simulink model "waterTankProcess_model_continuous_fullOrderObserver"  (R2017a)
settings: Solver=ode4  StartTime=0.0  StopTime=SIM_TIME  FixedStep=STEP_SIZE  RelTol=1e-3  EnableMultiTasking=on
values from neighbouring files (symbols this model uses):
  At = 0.785    [TwoTankSystem.m]
  Av0 = 0.0122    [TwoTankSystem.m]
  Av1 = 1.2*0.0122    (= 0.01464)    [TwoTankSystem.m]
  B = B(:,1:2)    [TwoTankSystem.m]
  C0 = 0.056    [TwoTankSystem.m]
  C1 = [0 kh 0 0;0 0 kt 0;0 0 0 kt]    [TwoTankSystem.m]
  Dv = 2.66    [TwoTankSystem.m]
  ka = 0.004    [TwoTankSystem.m]
  kh = 2    [TwoTankSystem.m]
  kt = 0.1    [TwoTankSystem.m]
  L = place(A',C',lambda_obs_des)'    [TwoTankSystem.m]
  L1 = place(A',C1',lambda_obs_des)'    [TwoTankSystem.m]
  T1 = 3000    [TwoTankSystem.m]
  T2 = 4000    [TwoTankSystem.m]
  Tc = 1500    [TwoTankSystem.m]
  Tc0 = 30    [TwoTankSystem.m]
  Tc1 = 20    [TwoTankSystem.m]
  Tv = 2200    [TwoTankSystem.m]
  Tw = 300    [TwoTankSystem.m]
  Tw0 = 60    [TwoTankSystem.m]
  Tw1 = 75    [TwoTankSystem.m]
  u0 = u0(1:2,1)    [TwoTankSystem.m]
  uc0 = 5    [TwoTankSystem.m]
  uc1 = 3.5    [TwoTankSystem.m]
  uw0 = 5    [TwoTankSystem.m]
  uw1 = 6.5    [TwoTankSystem.m]
  x0 = xFinal'    [TwoTankSystem.m]
  xhat0 = 1.0*x0-x0    [TwoTankSystem.m]
  Y0 = C*x0    [TwoTankSystem.m]
undefined symbols (not defined in the file or in its folder): A, C
settings Model: Creator=roga  LastModifiedBy=Roberto
settings DataIOCC: LimitDataPoints=on  SaveFinalState=on  SaveFormat=Array
settings OptimizationCC: LifeSpan=inf
settings DebuggingCC: UnderspecifiedInitializationDetection=Classic  MergeDetectMultiDrivingBlocksExec=none  SolverPrmCheckMsg=warning  StateNameClashWarn=warning  SFUnexpectedBacktrackingDiag=warning  SFNoUnconditionalDefaultTransitionDiag=warning  SFExecutionAtInitializationDiag=none
settings HardwareCC: ProdBitPerPointer=32  ProdBitPerSizeT=32  ProdBitPerPtrDiffT=32  ProdLargestAtomicFloat=None  ProdIntDivRoundTo=Undefined  ProdEndianess=Unspecified  ProdWordSize=32  ProdHWDeviceType=32-bit Generic
settings ModelReferenceCC: PropagateSignalLabelsOutOfModel=off
settings GRTTargetCC: TargetLangStandard=C89/C90 (ANSI)  GeneratePreprocessorConditionals=Disable all
settings ConfigComp: CovMetricSettings=dw  CovHtmlReporting=on  CovSaveCumulativeToWorkspaceVar=on  CovSaveSingleToWorkspaceVar=on  CovExternalEMLEnable=off

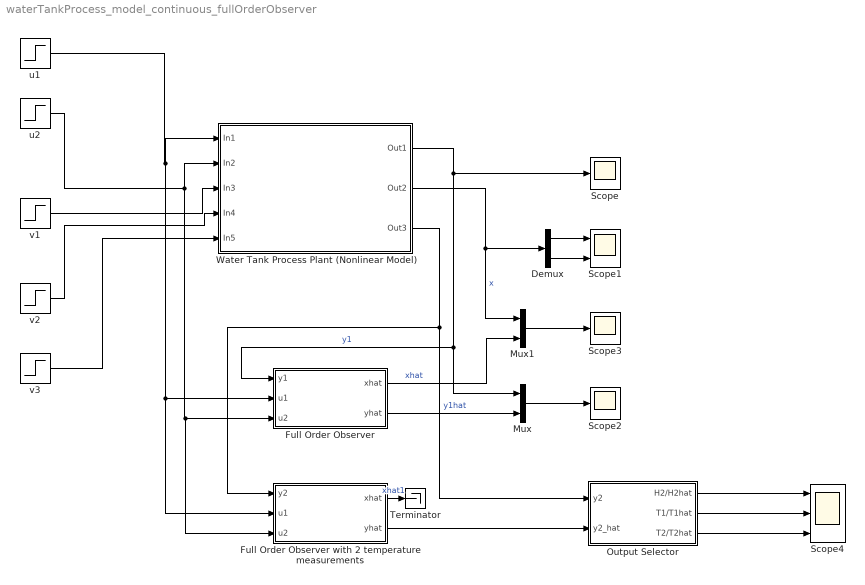
== system waterTankProcess_model_continuous_fullOrderObserver ==
  Demux : Demux  Outputs=2
  Full Order Observer : Subsystem
  Full Order Observer with 2 temperature measurements : Subsystem
  Mux : Mux  Inputs=2
  Mux1 : Mux  Inputs=2
  Output Selector : Subsystem
  Scope : Scope
  Scope1 : Scope  NumInputPorts=2
  Scope2 : Scope
  Scope3 : Scope
  Scope4 : Scope  NumInputPorts=3
  Terminator : Terminator
  Water Tank Process Plant (Nonlinear Model) : Subsystem
      mask Display:
      | port_label('output',1,'y_1','texmode','on')
      | port_label('output',2,'x','texmode','on')
      | port_label('output',3,'y_2','texmode','on')
      | port_label('input',1,'u_1','texmode','on')
      | port_label('input',2,'u_2','texmode','on')
      | port_label('input',3,'A_v','texmode','on')
      | port_label('input',4,'T_w','texmode','on')
      | port_label('input',5,'T_c','texmode','on')
  u1 : Step  Time=Tw  Before=uw0  After=uw1  SampleTime=0
  u2 : Step  Time=Tc  Before=uc0  After=uc1  SampleTime=0
  v1 : Step  Time=Tv  Before=Av0  After=Av1  SampleTime=0
  v2 : Step  Time=T1  Before=Tw0  After=Tw1  SampleTime=0
  v3 : Step  Time=T2  Before=Tc0  After=Tc1  SampleTime=0
  wires:
  Demux/1 -> Scope1/1
  Demux/2 -> Scope1/2
  u1/1 -> Full Order Observer with 2 temperature measurements/2(u1), Full Order Observer/2(u1), Water Tank Process Plant (Nonlinear Model)/1(In1)
  u2/1 -> Full Order Observer with 2 temperature measurements/3(u2), Full Order Observer/3(u2), Water Tank Process Plant (Nonlinear Model)/2(In2)
  v1/1 -> Water Tank Process Plant (Nonlinear Model)/3(In3)
  v2/1 -> Water Tank Process Plant (Nonlinear Model)/4(In4)
  v3/1 -> Water Tank Process Plant (Nonlinear Model)/5(In5)
  Water Tank Process Plant (Nonlinear Model)/2(Out2) -> Mux1/1, Demux/1  "x"
  Water Tank Process Plant (Nonlinear Model)/1(Out1) -> Mux/1, Full Order Observer/1(y1), Scope/1  "y1"
  Full Order Observer/2(yhat) -> Mux/2  "y1hat"
  Mux/1 -> Scope2/1
  Mux1/1 -> Scope3/1
  Full Order Observer/1(xhat) -> Mux1/2  "xhat"
  Water Tank Process Plant (Nonlinear Model)/3(Out3) -> Output Selector/1(y2), Full Order Observer with 2 temperature measurements/1(y2)
  Full Order Observer with 2 temperature measurements/2(yhat) -> Output Selector/2(y2_hat)
  Output Selector/1(H2/H2hat) -> Scope4/1
  Output Selector/2(T1/T1hat) -> Scope4/2
  Output Selector/3(T2/T2hat) -> Scope4/3
  Full Order Observer with 2 temperature measurements/1(xhat) -> Terminator/1  "xhat1"

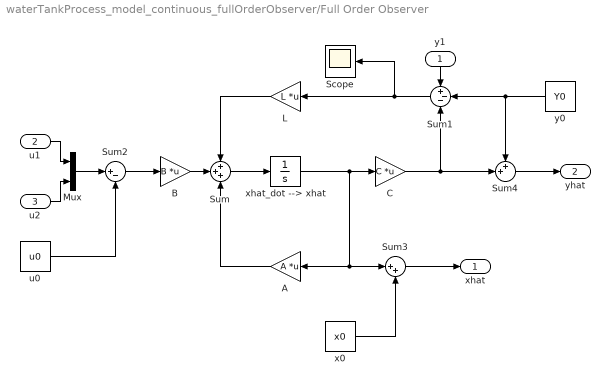
== system waterTankProcess_model_continuous_fullOrderObserver/Full Order Observer ==
  y1 : Inport
  u1 : Inport  Port=2
  u2 : Inport  Port=3
  A : Gain  Gain=A  Multiplication=Matrix(K*u) (u vector)
  B : Gain  Gain=B  Multiplication=Matrix(K*u) (u vector)
  C : Gain  Gain=C  Multiplication=Matrix(K*u) (u vector)
  L : Gain  Gain=L  Multiplication=Matrix(K*u) (u vector)
  Mux : Mux  Inputs=2
  Scope : Scope
  Sum : Sum  Inputs=+++
  Sum1 : Sum  Inputs=+--
  Sum2 : Sum  Inputs=|+-
  Sum3 : Sum  Inputs=|++
  Sum4 : Sum  Inputs=++|
  u0 : Constant  Value=u0
  x0 : Constant  Value=x0
  xhat_dot --> xhat : Integrator  InitialCondition=xhat0
  y0 : Constant  Value=Y0
  xhat : Outport
  yhat : Outport  Port=2
  wires:
  C/1 -> Sum4/2, Sum1/3
  Sum/1 -> xhat_dot --> xhat/1
  B/1 -> Sum/2
  A/1 -> Sum/3
  L/1 -> Sum/1
  Sum1/1 -> Scope/1, L/1
  xhat_dot --> xhat/1 -> C/1, Sum3/1, A/1
  u1/1 -> Mux/1
  u2/1 -> Mux/2
  y1/1 -> Sum1/1
  Sum2/1 -> B/1
  Mux/1 -> Sum2/1
  u0/1 -> Sum2/2
  y0/1 -> Sum4/1, Sum1/2
  Sum3/1 -> xhat/1
  x0/1 -> Sum3/2
  Sum4/1 -> yhat/1

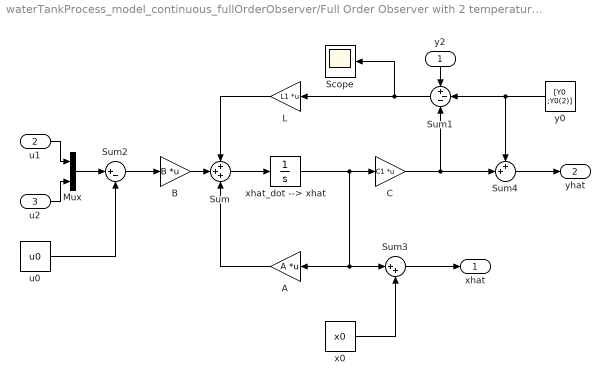
== system waterTankProcess_model_continuous_fullOrderObserver/Full Order Observer with 2 temperature measurements ==
  y2 : Inport
  u1 : Inport  Port=2
  u2 : Inport  Port=3
  A : Gain  Gain=A  Multiplication=Matrix(K*u) (u vector)
  B : Gain  Gain=B  Multiplication=Matrix(K*u) (u vector)
  C : Gain  Gain=C1  Multiplication=Matrix(K*u) (u vector)
  L : Gain  Gain=L1  Multiplication=Matrix(K*u) (u vector)
  Mux : Mux  Inputs=2
  Scope : Scope
  Sum : Sum  Inputs=+++
  Sum1 : Sum  Inputs=+--
  Sum2 : Sum  Inputs=|+-
  Sum3 : Sum  Inputs=|++
  Sum4 : Sum  Inputs=++|
  u0 : Constant  Value=u0
  x0 : Constant  Value=x0
  xhat_dot --> xhat : Integrator  InitialCondition=xhat0
  y0 : Constant  Value=[Y0 ;Y0(2)]
  xhat : Outport
  yhat : Outport  Port=2
  wires:
  Sum4/1 -> yhat/1
  x0/1 -> Sum3/2
  Sum3/1 -> xhat/1
  y0/1 -> Sum1/2, Sum4/1
  u0/1 -> Sum2/2
  Mux/1 -> Sum2/1
  Sum2/1 -> B/1
  y2/1 -> Sum1/1
  u2/1 -> Mux/2
  u1/1 -> Mux/1
  xhat_dot --> xhat/1 -> A/1, Sum3/1, C/1
  Sum1/1 -> L/1, Scope/1
  L/1 -> Sum/1
  A/1 -> Sum/3
  B/1 -> Sum/2
  Sum/1 -> xhat_dot --> xhat/1
  C/1 -> Sum1/3, Sum4/2

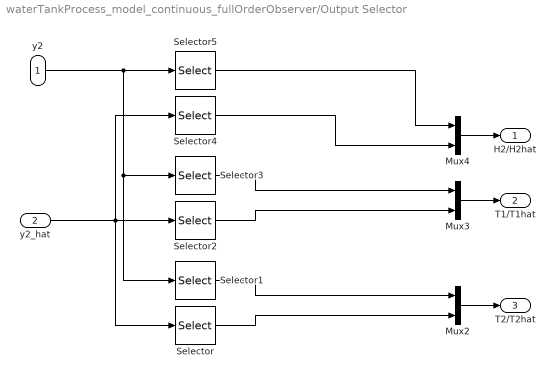
== system waterTankProcess_model_continuous_fullOrderObserver/Output Selector ==
  y2 : Inport
  y2_hat : Inport  Port=2
  Mux2 : Mux  Inputs=2
  Mux3 : Mux  Inputs=2
  Mux4 : Mux  Inputs=2
  Selector : Selector  InputPortWidth=3  IndexOptions=Index vector (dialog)  Indices=[3]  OutputSizes=1
  Selector1 : Selector  InputPortWidth=3  IndexOptions=Index vector (dialog)  Indices=[3]  OutputSizes=1
  Selector2 : Selector  InputPortWidth=3  IndexOptions=Index vector (dialog)  Indices=[2]  OutputSizes=1
  Selector3 : Selector  InputPortWidth=3  IndexOptions=Index vector (dialog)  Indices=[2]  OutputSizes=1
  Selector4 : Selector  InputPortWidth=3  IndexOptions=Index vector (dialog)  Indices=[1]  OutputSizes=1
  Selector5 : Selector  InputPortWidth=3  IndexOptions=Index vector (dialog)  Indices=[1]  OutputSizes=1
  H2/H2hat : Outport
  T1/T1hat : Outport  Port=2
  T2/T2hat : Outport  Port=3
  wires:
  Mux3/1 -> T1/T1hat/1
  Selector/1 -> Mux2/2
  Selector5/1 -> Mux4/1
  y2_hat/1 -> Selector4/1, Selector2/1, Selector/1
  Selector3/1 -> Mux3/1
  y2/1 -> Selector3/1, Selector1/1, Selector5/1
  Selector1/1 -> Mux2/1
  Mux2/1 -> T2/T2hat/1
  Selector2/1 -> Mux3/2
  Selector4/1 -> Mux4/2
  Mux4/1 -> H2/H2hat/1

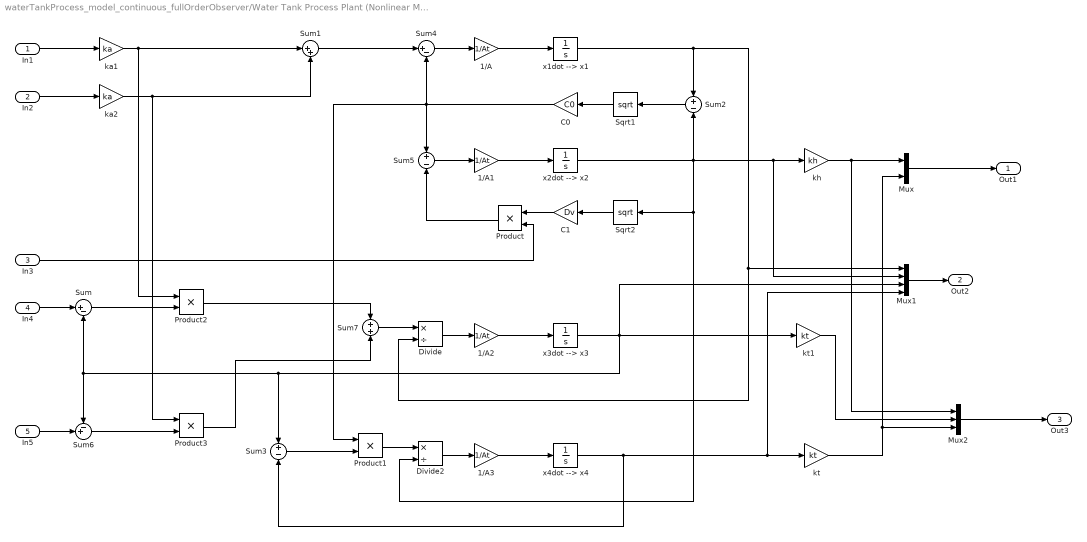
== system waterTankProcess_model_continuous_fullOrderObserver/Water Tank Process Plant (Nonlinear Model) ==
  In1 : Inport
  In2 : Inport  Port=2
  In3 : Inport  Port=3
  In4 : Inport  Port=4
  In5 : Inport  Port=5
  1/A{,1..3} (4 alike) : Gain  Gain=1/At
  C0 : Gain  Gain=C0
  C1 : Gain  Gain=Dv
  Divide : Product  Inputs=*/
  Divide2 : Product  Inputs=*/
  Mux : Mux  Inputs=2
  Mux1 : Mux
  Mux2 : Mux  Inputs=3
  Product{,1..3} (4 alike) : Product
  Sqrt1 : Sqrt  SaturateOnIntegerOverflow=on
  Sqrt2 : Sqrt  SaturateOnIntegerOverflow=on
  Sum : Sum  Inputs=|+-
  Sum1 : Sum  Inputs=|++
  Sum2 : Sum  Inputs=+-
  Sum3 : Sum  Inputs=+-
  Sum4 : Sum  Inputs=|+-
  Sum5 : Sum  Inputs=+-
  Sum6 : Sum  Inputs=-+|
  Sum7 : Sum
  ka1 : Gain  Gain=ka
  ka2 : Gain  Gain=ka
  kh : Gain  Gain=kh
  kt : Gain  Gain=kt
  kt1 : Gain  Gain=kt
  x1dot --> x1 : Integrator  InitialCondition=x0(1)  LimitOutput=on  LowerSaturationLimit=0
  x2dot --> x2 : Integrator  InitialCondition=x0(2)  LimitOutput=on  LowerSaturationLimit=0
  x3dot --> x3 : Integrator  InitialCondition=x0(3)
  x4dot --> x4 : Integrator  InitialCondition=x0(4)
  Out1 : Outport
  Out2 : Outport  Port=2
  Out3 : Outport  Port=3
  wires:
  Product1/1 -> Divide2/1
  In2/1 -> ka2/1
  Divide/1 -> 1/A2/1
  Sum6/1 -> Product3/2
  In4/1 -> Sum/1
  1/A1/1 -> x2dot --> x2/1
  Sum5/1 -> 1/A1/1
  Product/1 -> Sum5/2
  x1dot --> x1/1 -> Sum2/1, Mux1/1, Divide/2
  Sum/1 -> Product2/2
  C1/1 -> Product/1
  Sum3/1 -> Product1/2
  Sqrt2/1 -> C1/1
  1/A2/1 -> x3dot --> x3/1
  In1/1 -> ka1/1
  In3/1 -> Product/2
  kh/1 -> Mux2/1, Mux/1
  x4dot --> x4/1 -> Mux1/4, kt/1, Sum3/2
  C0/1 -> Sum4/2, Product1/1, Sum5/1
  1/A3/1 -> x4dot --> x4/1
  x2dot --> x2/1 -> Mux1/2, kh/1, Divide2/2, Sqrt2/1, Sum2/2
  Divide2/1 -> 1/A3/1
  Sum7/1 -> Divide/1
  In5/1 -> Sum6/2
  Product2/1 -> Sum7/1
  ka1/1 -> Product2/1, Sum1/1
  Product3/1 -> Sum7/2
  Mux/1 -> Out1/1
  ka2/1 -> Product3/1, Sum1/2
  kt/1 -> Mux2/3, Mux/2
  x3dot --> x3/1 -> kt1/1, Sum3/1, Sum6/1, Sum/2, Mux1/3
  1/A/1 -> x1dot --> x1/1
  Sum1/1 -> Sum4/1
  Mux1/1 -> Out2/1
  Sqrt1/1 -> C0/1
  Sum4/1 -> 1/A/1
  Sum2/1 -> Sqrt1/1
  Mux2/1 -> Out3/1
  kt1/1 -> Mux2/2
